simulink model "sensorMCUSlugsMKII"  (Simulink 6.6)
settings: Solver=FixedStepDiscrete  StartTime=0.0  StopTime=10.0  FixedStep=0.01  RelTol=1e-3
InitFcn:
  | mcuInit
values from neighbouring files (symbols this model uses):
  apSampleTime = 0.01    [mcuInit.m]
  T = 0.01    [mcuInit.m]
undefined symbols (not defined in the file or in its folder): accBiasRateLimit, accelXCutTemp, axTGain1, axTGain2, axTMean1, axTMean2, barAdjust, baroCutoff, baroCutTemp, baroOffset, baroScale, barTGain1, barTGain2, barTMean1, barTMean2, baseHeight, baseTemp, cubeAccelGain, cubeGyroGain, DiscIntNeverNeededParam, gaind, getCubeData, getGpsMainData, getMag, GS_location, gyroBiasRateLimit, lapseRate, lowRateSensorCutoff, magMeanTemp, magOffset, magScale, magTempK, mainSensorCutoff, maxDynPressure, param_acc, param_mag, pitAdjust, pitCutTemp, pitotOffset, pitotScale, pitTGain1, pitTGain2, pitTMean1, pitTMean2, polesd, powerOffset, powerScale, pressureSensorCutoff, q_quat, scheduleData, sensorMCUInit, spiSend, tempOffset, tempScale, u1, u2, updateAirData, updateAttitude, updateBias, updateDiagnosticFl ... (+14)
libraries: dsPICdrivers x38, simulink x14, aerolibutil x4, dspmtrx3 x2, aerolibconvert2 x2, SLUGS_Library x1
(part 2 of 4)

== system sensorMCUSlugsMKII/Position and Attitude Filter/GPS Update/Detect Change1 ==
  Data : Inport
  Abs1 : Abs  SampleTime=T
  Difference1 : simulink/Discrete/Difference  SystemSampleTime=-1  ICPrevInput=0.0  OutDataType=sfix(16)  OutScaling=2^-10  DoSatur=off
  Saturation1 : Saturate  UpperLimit=1  LowerLimit=0  SampleTime=T
  change? : Outport
  wires:
  Saturation1/1 -> change?/1
  Data/1 -> Difference1/1
  Abs1/1 -> Saturation1/1
  Difference1/1 -> Abs1/1

== system sensorMCUSlugsMKII/Position and Attitude Filter/GPS Update/Detect Change2 ==
  Data : Inport
  Abs1 : Abs  SampleTime=T
  Difference1 : simulink/Discrete/Difference  SystemSampleTime=-1  ICPrevInput=0.0  OutDataType=sfix(16)  OutScaling=2^-10  DoSatur=off
  Saturation1 : Saturate  UpperLimit=1  LowerLimit=0  SampleTime=T
  change? : Outport
  wires:
  Difference1/1 -> Abs1/1
  Abs1/1 -> Saturation1/1
  Data/1 -> Difference1/1
  Saturation1/1 -> change?/1

== system sensorMCUSlugsMKII/Position and Attitude Filter/Geod2LTP1/ECEF2LTP (UEN) ==
  ECEF coordinates : Inport
  "Long, Lat" : Inport  Port=2
  Deg2R : Gain  Gain=pi/180  SaturateOnIntegerOverflow=on
  Demux3 : Demux  Outputs=2
  From Body to Universal1 : Subsystem
  Product1 : Product  Multiplication=Matrix(*)  SaturateOnIntegerOverflow=on  InputSameDT=on
  Out : Outport
  wires:
  From Body to Universal1/1(DCM) -> Product1/1
  ECEF coordinates/1 -> Product1/2
  Deg2R/1 -> Demux3/1
  Demux3/1 -> From Body to Universal1/1(long)
  Demux3/2 -> From Body to Universal1/2(lat)
  Product1/1 -> Out/1
  "Long, Lat"/1 -> Deg2R/1

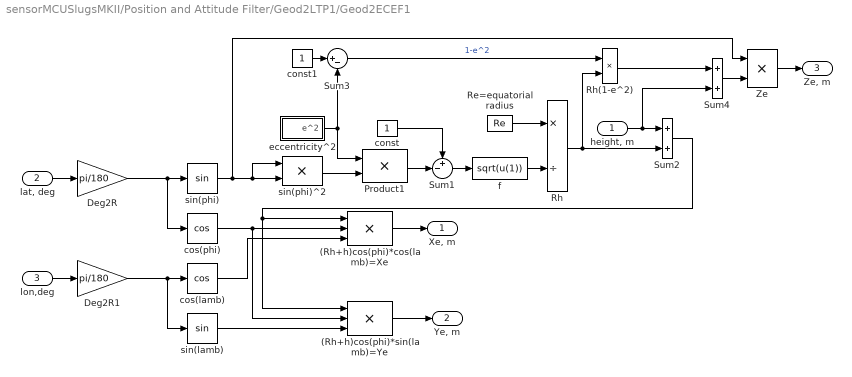
== system sensorMCUSlugsMKII/Position and Attitude Filter/Geod2LTP1/Geod2ECEF1 ==
  "height, m" : Inport
  "lat, deg" : Inport  Port=2
  lon,deg : Inport  Port=3
  (Rh+h)cos(phi)*cos(lamb)=Xe : Product  Inputs=3  OutDataTypeMode=single  SaturateOnIntegerOverflow=on  InputSameDT=on
  (Rh+h)cos(phi)*sin(lamb)=Ye : Product  Inputs=3  OutDataTypeMode=single  SaturateOnIntegerOverflow=on  InputSameDT=on
  Deg2R : Gain  Gain=pi/180  OutDataTypeMode=Specify via dialog  OutDataType=float('single')  SaturateOnIntegerOverflow=on
  Deg2R1 : Gain  Gain=pi/180  OutDataTypeMode=Specify via dialog  OutDataType=float('single')  SaturateOnIntegerOverflow=on
  Product1 : Product  SaturateOnIntegerOverflow=on  InputSameDT=on
  Re=equatorial radius : Constant  Value=Re  OutDataTypeMode=single
  Rh : Product  Inputs=*/  OutDataTypeMode=single  SaturateOnIntegerOverflow=on  InputSameDT=on
  Rh(1-e^2) : Product  OutDataTypeMode=single  SaturateOnIntegerOverflow=on  InputSameDT=on
  Sum1 : Sum  Inputs=+-|  SaturateOnIntegerOverflow=on  InputSameDT=on
  Sum2 : Sum  SaturateOnIntegerOverflow=on  InputSameDT=on
      settings: AttributesFormatString=Rh+h
  Sum3 : Sum  Inputs=|+-  SaturateOnIntegerOverflow=on  InputSameDT=on
  Sum4 : Sum  OutDataTypeMode=single  SaturateOnIntegerOverflow=on  InputSameDT=on
      settings: AttributesFormatString=(1-e^2)Rh+h
  Ze : Product  OutDataTypeMode=single  SaturateOnIntegerOverflow=on  InputSameDT=on
  const : Constant  OutDataTypeMode=single
  const1 : Constant  OutDataTypeMode=single
  cos(lamb) : Trigonometry  Operator=cos
  cos(phi) : Trigonometry  Operator=cos
  eccentricity^2 : Subsystem
  f : Fcn  Expr=sqrt(u(1))
  sin(lamb) : Trigonometry
  sin(phi) : Trigonometry
  sin(phi)^2 : Product  SaturateOnIntegerOverflow=on  InputSameDT=on
  "Xe, m " : Outport
  "Ye, m " : Outport  Port=2
  "Ze, m " : Outport  Port=3
  wires:
  (Rh+h)cos(phi)*sin(lamb)=Ye/1 -> "Ye, m "/1
  (Rh+h)cos(phi)*cos(lamb)=Xe/1 -> "Xe, m "/1
  Sum2/1 -> (Rh+h)cos(phi)*cos(lamb)=Xe/1, (Rh+h)cos(phi)*sin(lamb)=Ye/1
  Deg2R1/1 -> sin(lamb)/1, cos(lamb)/1
  Deg2R/1 -> sin(phi)/1, cos(phi)/1
  Ze/1 -> "Ze, m "/1
  sin(lamb)/1 -> (Rh+h)cos(phi)*sin(lamb)=Ye/3
  cos(lamb)/1 -> (Rh+h)cos(phi)*cos(lamb)=Xe/3
  cos(phi)/1 -> (Rh+h)cos(phi)*sin(lamb)=Ye/2, (Rh+h)cos(phi)*cos(lamb)=Xe/2
  lon,deg/1 -> Deg2R1/1
  Sum4/1 -> Ze/2
  Rh(1-e^2)/1 -> Sum4/1
  Sum3/1 -> Rh(1-e^2)/1  "1-e^2"
  const1/1 -> Sum3/1
  sin(phi)^2/1 -> Product1/2
  eccentricity^2/1(e^2) -> Sum3/2, Product1/1
  "height, m"/1 -> Sum2/1, Sum4/2
  const/1 -> Sum1/1
  Sum1/1 -> f/1
  Product1/1 -> Sum1/2
  Rh/1 -> Rh(1-e^2)/2, Sum2/2
  Re=equatorial radius/1 -> Rh/1
  f/1 -> Rh/2
  sin(phi)/1 -> Ze/1, sin(phi)^2/2, sin(phi)^2/1
  "lat, deg"/1 -> Deg2R/1

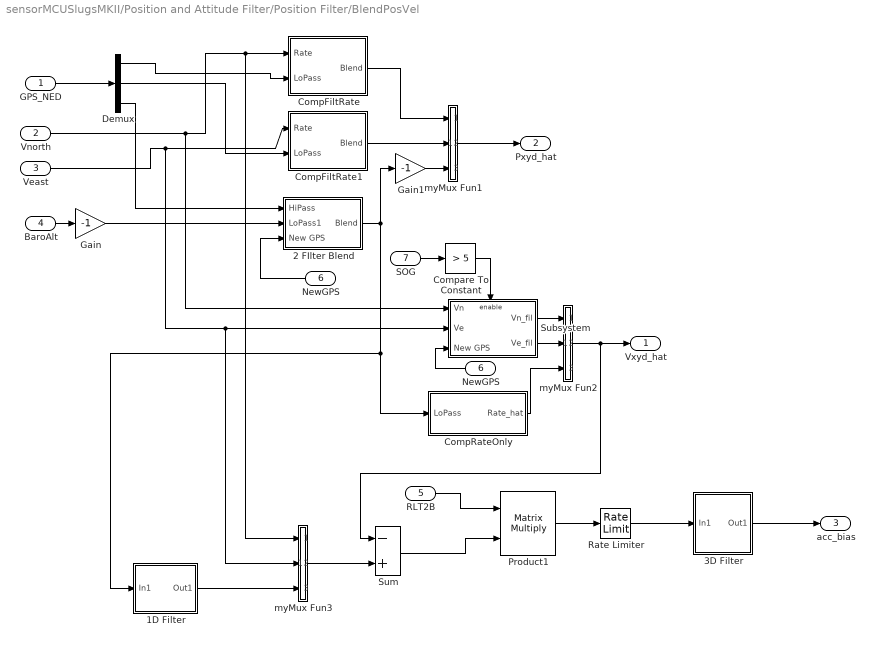
== system sensorMCUSlugsMKII/Position and Attitude Filter/Position Filter/BlendPosVel ==
  GPS_NED : Inport
  Vnorth : Inport  Port=2
  Veast : Inport  Port=3
  BaroAlt : Inport  Port=4
  RLT2B : Inport  Port=5
  NewGPS : Inport  Orientation=left  Port=6
  SOG : Inport  Port=7
  1D Filter : Subsystem  AncestorBlock=SLUGS_Library/Singnal Routing & Conditioning/3D Filter  RTWFcnName=TustinFilter3D  mask{zval=[0], pval=-50, kval=1, TSample=apSampleTime}
      mask prompts: zval "Zeros"; pval "Poles"; kval "Gains"; TSample "Sample Time"
      settings: RTWFcnNameOpts=User specified  RTWFileNameOpts=Use function name
      mask Display:
      | droots(zval,pval,kval)
      | port_label('input',1,'1D')
  2 FIlter Blend : Subsystem
  3D Filter : Subsystem  AncestorBlock=SLUGS_Library/Singnal Routing & Conditioning/3D Filter  RTWFcnName=TustinFilter3D  mask{zval=[], pval=[0], kval=1, TSample=0.01}
      mask prompts: zval "Zeros"; pval "Poles"; kval "Gains"; TSample "Sample Time"
      settings: RTWFcnNameOpts=User specified  RTWFileNameOpts=Use function name
      mask Display:
      | droots(zval,pval,kval)
      | port_label('input',1,'3D')
  CompFiltRate : Subsystem  mask{omega=xCutoff, T=apSampleTime}
      mask prompts: omega "Cutoff Freq (rad/sec)"; T "Sample Time"
  CompFiltRate1 : Subsystem  mask{omega=yCutoff, T=apSampleTime}
      mask prompts: omega "Cutoff Freq (rad/sec)"; T "Sample Time"
  CompRateOnly : Subsystem  mask{omega=vzCutoff, T=apSampleTime}
      mask prompts: omega "Cutoff Freq (rad/sec)"; T "Sample Time"
  Compare To Constant : simulink/Logic and Bit Operations/Compare To Constant  SystemSampleTime=-1  relop=>  const=5  LogicOutDataTypeMode=uint8  ZeroCross=off
  Demux : Demux  Outputs=3
  Gain : Gain  Gain=-1
  Gain1 : Gain  Gain=-1
  "NewGPS " : InportShadow  Orientation=left  Port=6  LatchByCopyingInsideSignal=off
  Product1 : Product  Multiplication=Matrix(*)  RndMeth=Zero
  Rate Limiter : RateLimiter  RisingSlewLimit=accBiasRateLimit  FallingSlewLimit=-accBiasRateLimit  SampleTimeMode=inherited
  Subsystem : Subsystem
  Sum : Sum  Inputs=-+  OutDataTypeMode=single
  myMux Fun1 : Stateflow chart
  myMux Fun2 : Stateflow chart
  myMux Fun3 : Stateflow chart
  Vxyd_hat : Outport
  Pxyd_hat : Outport  Port=2
  acc_bias : Outport  Port=3
  wires:
  Rate Limiter/1 -> 3D Filter/1(In1)
  3D Filter/1(Out1) -> acc_bias/1
  Sum/1 -> Product1/2
  myMux Fun3/1(y) -> Sum/2
  1D Filter/1(Out1) -> myMux Fun3/3(u3)
  Product1/1 -> Rate Limiter/1
  RLT2B/1 -> Product1/1
  CompRateOnly/1(Rate_hat) -> myMux Fun2/3(u3)
  Subsystem/2(Ve_fil) -> myMux Fun2/2(u2)
  Subsystem/1(Vn_fil) -> myMux Fun2/1(u1)
  Gain/1 -> 2 FIlter Blend/2(LoPass1)
  myMux Fun1/1(y) -> Pxyd_hat/1
  2 FIlter Blend/1(Blend) -> 1D Filter/1(In1), CompRateOnly/1(LoPass), Gain1/1
  CompFiltRate/1(Blend) -> myMux Fun1/1(u1)
  CompFiltRate1/1(Blend) -> myMux Fun1/2(u2)
  Demux/3 -> 2 FIlter Blend/1(HiPass)
  BaroAlt/1 -> Gain/1
  Demux/2 -> CompFiltRate1/2(LoPass)
  Demux/1 -> CompFiltRate/2(LoPass)
  Veast/1 -> myMux Fun3/2(u2), Subsystem/2(Ve), CompFiltRate1/1(Rate)
  Vnorth/1 -> CompFiltRate/1(Rate), myMux Fun3/1(u1), Subsystem/1(Vn)
  GPS_NED/1 -> Demux/1
  Gain1/1 -> myMux Fun1/3(u3)
  myMux Fun2/1(y) -> Vxyd_hat/1, Sum/1
  NewGPS/1 -> Subsystem/3(New GPS)
  Compare To Constant/1 -> Subsystem/Enable
  SOG/1 -> Compare To Constant/1
  "NewGPS "/1 -> 2 FIlter Blend/3(New GPS)

== system sensorMCUSlugsMKII/Sensor Data/Sensor Suite/Compute CPU Load ==
  Calculus Time Step : dsPICdrivers/OTHERS/Calculus Time Step  Tag=dsPIC_CalculusTimeStep  SampleTime=0.01  PR1chk=on
  Data Type Conversion1 : DataTypeConversion  OutDataTypeMode=single
  Data Type Conversion12 : DataTypeConversion  OutDataTypeMode=uint8
  Data Type Conversion2 : DataTypeConversion  OutDataTypeMode=single
  Divide : Product  Inputs=*/  OutDataTypeMode=double  OutScaling=2^-10
  Gain : Gain  Gain=100
  Rounding Function : Rounding
  Load (%) : Outport
  wires:
  Calculus Time Step/1 -> Data Type Conversion2/1
  Calculus Time Step/2 -> Data Type Conversion1/1
  Divide/1 -> Gain/1
  Rounding Function/1 -> Data Type Conversion12/1
  Data Type Conversion1/1 -> Divide/2
  Data Type Conversion2/1 -> Divide/1
  Data Type Conversion12/1 -> Load (%)/1
  Gain/1 -> Rounding Function/1

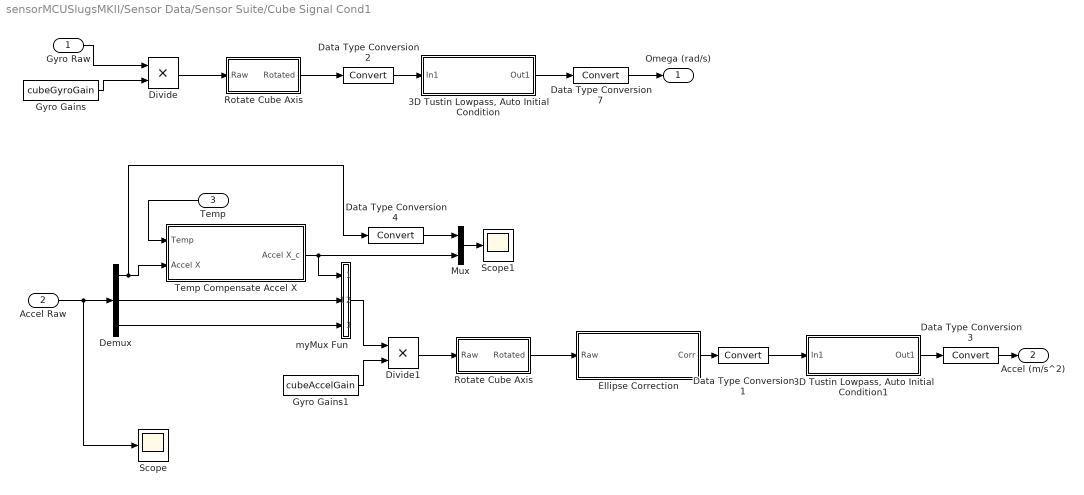
== system sensorMCUSlugsMKII/Sensor Data/Sensor Suite/Cube Signal Cond1 ==
  Gyro Raw : Inport
  Accel Raw : Inport  Port=2
  Temp : Inport  Orientation=left  Port=3
  "3D Tustin Lowpass, Auto Initial Condition" : Subsystem  mask(Tustin1stOrderLowpassAutoInitialCondition){f=mainSensorCutoff, T=T}
      mask prompts: f "Lowpass Frequency"; T "Sample Time"
      mask help: Takes a 3db rolloff frequency (in Hz, NOT radians/s) and a sample time. Performs a symbolic Tustin conversion and implements in a discrete filter. The initial output of the filter is set by the first sample.
      mask Help: Enter the desired 3db rolloff frequency in Hz and the sample time. Initial conditions are sampled automatically.
      mask Display: fprintf('%.2f Hz lowpass (3D)',f)
  "3D Tustin Lowpass, Auto Initial Condition1" : Subsystem  mask(Tustin1stOrderLowpassAutoInitialCondition){f=mainSensorCutoff, T=T}
      mask prompts: f "Lowpass Frequency"; T "Sample Time"
      mask help: Takes a 3db rolloff frequency (in Hz, NOT radians/s) and a sample time. Performs a symbolic Tustin conversion and implements in a discrete filter. The initial output of the filter is set by the first sample.
      mask Help: Enter the desired 3db rolloff frequency in Hz and the sample time. Initial conditions are sampled automatically.
      mask Display: fprintf('%.2f Hz lowpass (3D)',f)
  Data Type Conversion1 : DataTypeConversion  OutDataTypeMode=double
  Data Type Conversion2 : DataTypeConversion  OutDataTypeMode=double
  Data Type Conversion3 : DataTypeConversion  OutDataTypeMode=single
  Data Type Conversion4 : DataTypeConversion  OutDataTypeMode=single
  Data Type Conversion7 : DataTypeConversion  OutDataTypeMode=single
  Demux : Demux  Outputs=3
  Divide : Product  OutDataTypeMode=single  OutScaling=2^-10
  Divide1 : Product  OutDataTypeMode=single  OutScaling=2^-10
  Ellipse Correction : Subsystem  AncestorBlock=SLUGS_Library/Singnal Routing & Conditioning/Ellipse Correction  mask{param=param_acc}
      mask prompts: param "parameter (struct)"
      mask help: Applies the correction from the ellipse algorithm to the raw data being sent through the block. The block expects a 3x1 input vector, and will return a 3x1 output vector. The parameter constant should be a struct with param.xo .yo and .zo being the offsets, param.a .b and .c being the scale factors, and param.phi .rho and .lambda being the angle non-orthogonality (in degrees).
      mask Display:
      | text(0.2,0.85,'Ellipse Correction')
      | port_label('input',1,'RAW')
      | port_label('output',1,'CORR')
  Gyro Gains : Constant  Value=cubeGyroGain  OutDataTypeMode=single
  Gyro Gains1 : Constant  Value=cubeAccelGain  OutDataTypeMode=single
  Mux : Mux  Inputs=2
  Rotate Cube Axis : Subsystem
  "Rotate Cube Axis " : Subsystem
  Scope : Scope
      settings: YMin=-22.5  YMax=15  SaveName=ScopeData13
  Scope1 : Scope
      settings: YMin=-225  YMax=275  SaveName=ScopeData15
  Temp Compensate Accel X : Subsystem
  myMux Fun : Stateflow chart
  Omega (rad/s) : Outport
  Accel (m/s^2) : Outport  Port=2
  wires:
  Data Type Conversion4/1 -> Mux/1
  Mux/1 -> Scope1/1
  Demux/2 -> myMux Fun/2(u2)
  Gyro Gains/1 -> Divide/2
  Divide/1 -> Rotate Cube Axis/1(Raw)
  Divide1/1 -> "Rotate Cube Axis "/1(Raw)
  "Rotate Cube Axis "/1(Rotated) -> Ellipse Correction/1(Raw)
  Gyro Gains1/1 -> Divide1/2
  Gyro Raw/1 -> Divide/1
  Data Type Conversion2/1 -> "3D Tustin Lowpass, Auto Initial Condition"/1(In1)
  "3D Tustin Lowpass, Auto Initial Condition"/1(Out1) -> Data Type Conversion7/1
  Data Type Conversion7/1 -> Omega (rad/s)/1
  Rotate Cube Axis/1(Rotated) -> Data Type Conversion2/1
  Data Type Conversion1/1 -> "3D Tustin Lowpass, Auto Initial Condition1"/1(In1)
  "3D Tustin Lowpass, Auto Initial Condition1"/1(Out1) -> Data Type Conversion3/1
  Data Type Conversion3/1 -> Accel (m/s^2)/1
  Ellipse Correction/1(Corr) -> Data Type Conversion1/1
  Temp/1 -> Temp Compensate Accel X/1(Temp)
  Demux/3 -> myMux Fun/3(u3)
  Temp Compensate Accel X/1(Accel X_c) -> Mux/2, myMux Fun/1(u1)
  Demux/1 -> Data Type Conversion4/1, Temp Compensate Accel X/2(Accel X)
  Accel Raw/1 -> Scope/1, Demux/1
  myMux Fun/1(y) -> Divide1/1

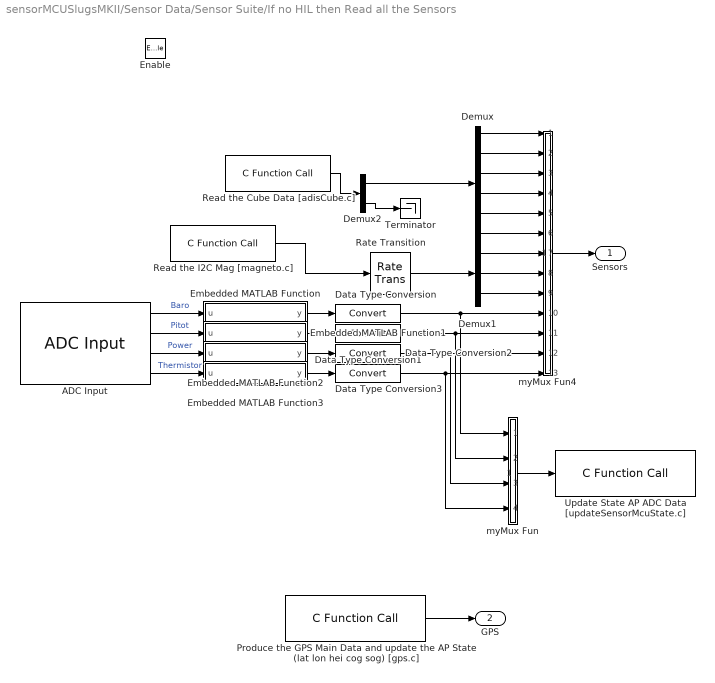
== system sensorMCUSlugsMKII/Sensor Data/Sensor Suite/If no HIL then Read all the Sensors ==
  Enable : EnablePort
  ADC Input : dsPICdrivers/Peripheral I//O/ADC Input  Tag=dsPIC_ADC  Priority=5  ADC_TYPE=12 bits  ADC_MODE=Continuous sampling & get last channel value  NbrSampleStep=4  VoltRefpopup="AVdd  -  AVss"  OutFormatBitspopup=0000 dddd dddd dddd : Integer  InterruptPriority=6  ANCHANNELS=[8 9 10 11]  MaxName=ANmax = 4095  Rin=200  ADCS=63  SAMC=31  Temperature=25  DMAChannel=1  SampleTime=.01  Status="OK  |  Tsmp=2.480e-005 |  T/Channel=3.600e-005 |  Tall=5.760e-004"  SSRC=auto convert
  Data Type Conversion{,1..3} (4 alike) : DataTypeConversion  OutDataTypeMode=int16
  Demux : Demux  Outputs=6
  Demux1 : Demux  Outputs=3
  Demux2 : Demux  Outputs=[6 1]
  Embedded MATLAB Function : Stateflow chart
  Embedded MATLAB Function1 : Stateflow chart
  Embedded MATLAB Function2 : Stateflow chart
  Embedded MATLAB Function3 : Stateflow chart
  Produce the GPS Main Data and update the AP State (lat lon hei cog sog) [gps.c] : dsPICdrivers/OTHERS/C Function Call  Tag=dsPIC_dsPIC_CFunctionCall  fctName='getGpsMainData'  INPUT_SIZE=1  INPUT1=--  INPUT2=--  INPUT3=--  OUTPUT_SIZE=5  OUTPUT1=real32  SampleTime=.01  InputType=[ ]  OutputType=[ 7 ]  FctDeclaration=extern void getGpsMainData(real32_T* y1);  FctCall=getGpsMainData(*%y1);  OrderingInOutPopup=None
  Rate Transition : RateTransition  OutPortSampleTime=0.01
  Read the Cube Data [adisCube.c] : dsPICdrivers/OTHERS/C Function Call  Tag=dsPIC_dsPIC_CFunctionCall  fctName='getCubeData'  INPUT_SIZE=1  INPUT1=--  INPUT2=--  INPUT3=--  OUTPUT_SIZE=7  OUTPUT1=int16  SampleTime=.01  InputType=[ ]  OutputType=[ 3 ]  FctDeclaration=extern void getCubeData(int16_T* y1);  FctCall=getCubeData(*%y1);  OrderingInOutPopup=None
  Read the I2C Mag [magneto.c] : dsPICdrivers/OTHERS/C Function Call  Tag=dsPIC_dsPIC_CFunctionCall  fctName='getMag'  INPUT_SIZE=1  INPUT1=--  INPUT2=--  INPUT3=--  OUTPUT_SIZE=3  OUTPUT1=int16  SampleTime=.01  InputType=[ ]  OutputType=[ 3 ]  FctDeclaration=extern void getMag(int16_T* y1);  FctCall=getMag(*%y1);  OrderingInOutPopup=None
  Terminator : Terminator
  Update State AP ADC Data [updateSensorMcuState.c] : dsPICdrivers/OTHERS/C Function Call  Tag=dsPIC_dsPIC_CFunctionCall  fctName='updateRawADCData'  INPUT_SIZE=4  INPUT1=int16  INPUT2=--  INPUT3=--  OUTPUT_SIZE=1  OUTPUT1=--  SampleTime=.01  InputType=[ 3 ]  OutputType=[ ]  FctDeclaration=extern void updateRawADCData(int16_T* u1);  FctCall=updateRawADCData(*%u1);  OrderingInOutPopup=None
  myMux Fun : Stateflow chart
  myMux Fun4 : Stateflow chart
  Sensors : Outport
  GPS : Outport  Port=2
  wires:
  myMux Fun4/1(y) -> Sensors/1
  Demux2/1 -> Demux/1
  Read the I2C Mag [magneto.c]/1 -> Rate Transition/1
  Demux/1 -> myMux Fun4/1(u1)
  Demux/2 -> myMux Fun4/2(u2)
  Demux/3 -> myMux Fun4/3(u3)
  Demux/4 -> myMux Fun4/4(u4)
  Demux/5 -> myMux Fun4/5(u5)
  Demux/6 -> myMux Fun4/6(u6)
  Demux1/1 -> myMux Fun4/7(u7)
  Demux1/2 -> myMux Fun4/8(u8)
  Demux1/3 -> myMux Fun4/9(u9)
  ADC Input/1 -> Embedded MATLAB Function/1(u)  "Baro"
  ADC Input/2 -> Embedded MATLAB Function1/1(u)  "Pitot"
  ADC Input/3 -> Embedded MATLAB Function2/1(u)  "Power"
  ADC Input/4 -> Embedded MATLAB Function3/1(u)  "Thermistor"
  myMux Fun/1(y) -> Update State AP ADC Data [updateSensorMcuState.c]/1
  Rate Transition/1 -> Demux1/1
  Data Type Conversion/1 -> myMux Fun4/10(u10), myMux Fun/1(u1)
  Data Type Conversion1/1 -> myMux Fun4/11(u11), myMux Fun/2(u2)
  Data Type Conversion2/1 -> myMux Fun4/12(u12), myMux Fun/3(u3)
  Data Type Conversion3/1 -> myMux Fun4/13(u13), myMux Fun/4(u4)
  Produce the GPS Main Data and update the AP State (lat lon hei cog sog) [gps.c]/1 -> GPS/1
  Embedded MATLAB Function/1(y) -> Data Type Conversion/1
  Embedded MATLAB Function1/1(y) -> Data Type Conversion1/1
  Embedded MATLAB Function2/1(y) -> Data Type Conversion2/1
  Embedded MATLAB Function3/1(y) -> Data Type Conversion3/1
  Read the Cube Data [adisCube.c]/1 -> Demux2/1
  Demux2/2 -> Terminator/1

== system sensorMCUSlugsMKII/Sensor Data/Sensor Suite/If no HIL then update Air Data ==
  AirData : Inport
  Enable : EnablePort
  Update the Air Calibrated Data [updateSensorMcuState.c] : dsPICdrivers/OTHERS/C Function Call  Tag=dsPIC_dsPIC_CFunctionCall  fctName='updateAirData'  INPUT_SIZE=3  INPUT1=real32  INPUT2=--  INPUT3=--  OUTPUT_SIZE=1  OUTPUT1=--  SampleTime=.01  InputType=[ 7 ]  OutputType=[ ]  FctDeclaration=extern void updateAirData(real32_T* u1);  FctCall=updateAirData(*%u1);  OrderingInOutPopup=None
  wires:
  AirData/1 -> Update the Air Calibrated Data [updateSensorMcuState.c]/1

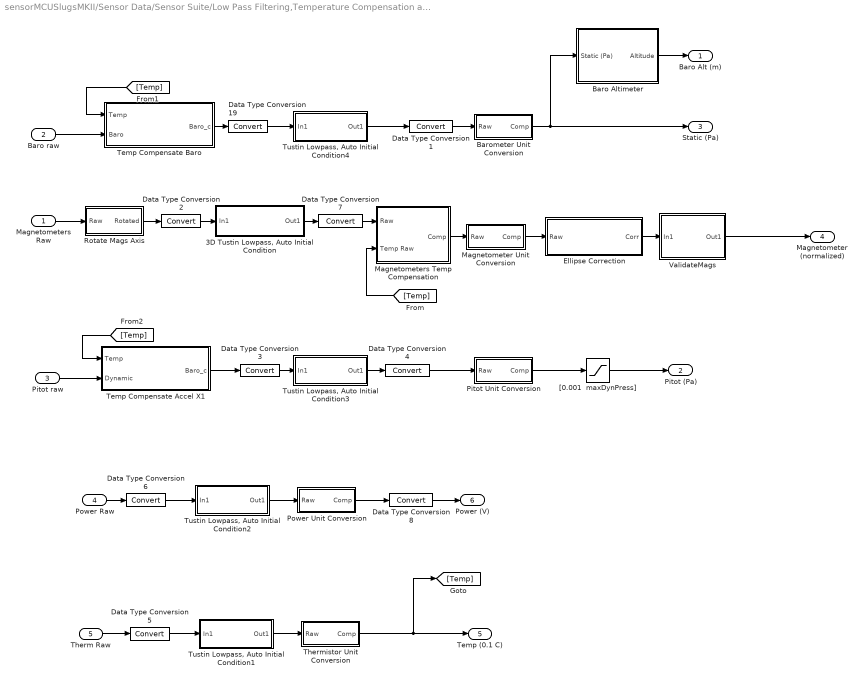
== system sensorMCUSlugsMKII/Sensor Data/Sensor Suite/Low Pass Filtering,Temperature Compensation and Calibration1 ==
  Magnetometers Raw : Inport
  Baro raw : Inport  Port=2
  Pitot raw : Inport  Port=3
  Power Raw : Inport  Port=4
  Therm Raw : Inport  Port=5
  "3D Tustin Lowpass, Auto Initial Condition" : Subsystem  mask(Tustin1stOrderLowpassAutoInitialCondition){f=mainSensorCutoff, T=T}
      mask prompts: f "Lowpass Frequency"; T "Sample Time"
      mask help: Takes a 3db rolloff frequency (in Hz, NOT radians/s) and a sample time. Performs a symbolic Tustin conversion and implements in a discrete filter. The initial output of the filter is set by the first sample.
      mask Help: Enter the desired 3db rolloff frequency in Hz and the sample time. Initial conditions are sampled automatically.
      mask Display: fprintf('%.2f Hz lowpass (3D)',f)
  Baro Altimeter : Subsystem
  Barometer Unit Conversion : Subsystem  mask{bias=baroOffset, gains=baroScale}
      mask prompts: bias "Initial Bias"; gains "Initial Gains"
      mask help: Convert Analog readings to units
  Data Type Conversion1 : DataTypeConversion  OutDataTypeMode=single
  Data Type Conversion{2..3,5..6,19} (5 alike) : DataTypeConversion  OutDataTypeMode=double
  Data Type Conversion4 : DataTypeConversion  OutDataTypeMode=single
  Data Type Conversion7 : DataTypeConversion  OutDataTypeMode=single
  Data Type Conversion8 : DataTypeConversion  OutDataTypeMode=uint16
  Ellipse Correction : Subsystem  AncestorBlock=SLUGS_Library/Singnal Routing & Conditioning/Ellipse Correction  mask{param=param_mag}
      mask prompts: param "parameter (struct)"
      mask help: Applies the correction from the ellipse algorithm to the raw data being sent through the block. The block expects a 3x1 input vector, and will return a 3x1 output vector. The parameter constant should be a struct with param.xo .yo and .zo being the offsets, param.a .b and .c being the scale factors, and param.phi .rho and .lambda being the angle non-orthogonality (in degrees).
      mask Display:
      | text(0.2,0.85,'Ellipse Correction')
      | port_label('input',1,'RAW')
      | port_label('output',1,'CORR')
  Magnetometer Unit Conversion : Subsystem  mask{bias=magOffset, gains=magScale}
      mask prompts: bias "Initial Bias"; gains "Initial Gains"
      mask help: Convert Analog readings to units
  Magnetometers Temp Compensation : Subsystem  mask{alpha=magTempK, tempMean=magMeanTemp}
      mask prompts: alpha "Tempearature Coeficient (K_t)"; tempMean "Calibration Temperature Mean (T_avg)"
      mask help:
      | This block implements a temperature compensation. It implmements the following equation:
      |
      | M_tc = M_raw - K_t(T - T_avg)
  Pitot Unit Conversion : Subsystem  mask{bias=pitotOffset, gains=pitotScale}
      mask prompts: bias "Initial Bias"; gains "Initial Gains"
      mask help: Convert Analog readings to units
  Power Unit Conversion : Subsystem  mask{bias=powerOffset, gains=powerScale}
      mask prompts: bias "Initial Bias"; gains "Initial Gains"
      mask help: Convert Analog readings to units
  Rotate Mags Axis : Subsystem
  Temp Compensate Accel X1 : Subsystem
  Temp Compensate Baro : Subsystem
  Thermistor Unit Conversion : Subsystem  mask{bias=tempOffset, gains=tempScale}
      mask prompts: bias "Initial Bias"; gains "Initial Gains"
      mask help: Convert Analog readings to units
  "Tustin Lowpass, Auto Initial Condition1" : Subsystem  mask(Tustin1stOrderLowpassAutoInitialCondition){f=lowRateSensorCutoff, T=T}
      mask prompts: f "Lowpass Frequency"; T "Sample Time"
      mask help: Takes a 3db rolloff frequency (in Hz, NOT radians/s) and a sample time. Performs a symbolic Tustin conversion and implements in a discrete filter. The initial output of the filter is set by the first sample.
      mask Help: Enter the desired 3db rolloff frequency in Hz and the sample time. Initial conditions are sampled automatically.
      mask Display: fprintf('%.2f Hz lowpass',f)
  "Tustin Lowpass, Auto Initial Condition2" : Subsystem  mask(Tustin1stOrderLowpassAutoInitialCondition){f=lowRateSensorCutoff, T=T}
      mask prompts: f "Lowpass Frequency"; T "Sample Time"
      mask help: Takes a 3db rolloff frequency (in Hz, NOT radians/s) and a sample time. Performs a symbolic Tustin conversion and implements in a discrete filter. The initial output of the filter is set by the first sample.
      mask Help: Enter the desired 3db rolloff frequency in Hz and the sample time. Initial conditions are sampled automatically.
      mask Display: fprintf('%.2f Hz lowpass',f)
  "Tustin Lowpass, Auto Initial Condition3" : Subsystem  mask(Tustin1stOrderLowpassAutoInitialCondition){f=pressureSensorCutoff, T=T}
      mask prompts: f "Lowpass Frequency"; T "Sample Time"
      mask help: Takes a 3db rolloff frequency (in Hz, NOT radians/s) and a sample time. Performs a symbolic Tustin conversion and implements in a discrete filter. The initial output of the filter is set by the first sample.
      mask Help: Enter the desired 3db rolloff frequency in Hz and the sample time. Initial conditions are sampled automatically.
      mask Display: fprintf('%.2f Hz lowpass',f)
  "Tustin Lowpass, Auto Initial Condition4" : Subsystem  mask(Tustin1stOrderLowpassAutoInitialCondition){f=pressureSensorCutoff, T=T}
      mask prompts: f "Lowpass Frequency"; T "Sample Time"
      mask help: Takes a 3db rolloff frequency (in Hz, NOT radians/s) and a sample time. Performs a symbolic Tustin conversion and implements in a discrete filter. The initial output of the filter is set by the first sample.
      mask Help: Enter the desired 3db rolloff frequency in Hz and the sample time. Initial conditions are sampled automatically.
      mask Display: fprintf('%.2f Hz lowpass',f)
  ValidateMags : Subsystem
  "[0.001  maxDynPress]" : Saturate  UpperLimit=maxDynPressure  LowerLimit=0.001
  Baro Alt (m) : Outport
  Pitot (Pa) : Outport  Port=2
  Static (Pa) : Outport  Port=3
  Magnetometer (normalized) : Outport  Port=4
  Temp (0.1 C) : Outport  Port=5
  Power (V) : Outport  Port=6
  wires:
  Data Type Conversion2/1 -> "3D Tustin Lowpass, Auto Initial Condition"/1(In1)
  "3D Tustin Lowpass, Auto Initial Condition"/1(Out1) -> Data Type Conversion7/1
  "Tustin Lowpass, Auto Initial Condition1"/1(Out1) -> Thermistor Unit Conversion/1(Raw)
  "[0.001  maxDynPress]"/1 -> Pitot (Pa)/1
  Data Type Conversion19/1 -> "Tustin Lowpass, Auto Initial Condition4"/1(In1)
  Data Type Conversion3/1 -> "Tustin Lowpass, Auto Initial Condition3"/1(In1)
  "Tustin Lowpass, Auto Initial Condition3"/1(Out1) -> Data Type Conversion4/1
  Data Type Conversion5/1 -> "Tustin Lowpass, Auto Initial Condition1"/1(In1)
  Therm Raw/1 -> Data Type Conversion5/1
  Barometer Unit Conversion/1(Comp) -> Static (Pa)/1, Baro Altimeter/1(Static (Pa))
  Magnetometers Raw/1 -> Rotate Mags Axis/1(Raw)
  Data Type Conversion4/1 -> Pitot Unit Conversion/1(Raw)
  Data Type Conversion7/1 -> Magnetometers Temp Compensation/1(Raw)
  Magnetometers Temp Compensation/1(Comp) -> Magnetometer Unit Conversion/1(Raw)
  [Temp] -> Magnetometers Temp Compensation/2(Temp Raw)
  "Tustin Lowpass, Auto Initial Condition4"/1(Out1) -> Data Type Conversion1/1
  Data Type Conversion1/1 -> Barometer Unit Conversion/1(Raw)
  Thermistor Unit Conversion/1(Comp) -> Temp (0.1 C)/1, [Temp]
  Data Type Conversion6/1 -> "Tustin Lowpass, Auto Initial Condition2"/1(In1)
  Power Raw/1 -> Data Type Conversion6/1
  "Tustin Lowpass, Auto Initial Condition2"/1(Out1) -> Power Unit Conversion/1(Raw)
  Data Type Conversion8/1 -> Power (V)/1
  Baro Altimeter/1(Altitude) -> Baro Alt (m)/1
  Pitot Unit Conversion/1(Comp) -> "[0.001  maxDynPress]"/1
  Power Unit Conversion/1(Comp) -> Data Type Conversion8/1
  Magnetometer Unit Conversion/1(Comp) -> Ellipse Correction/1(Raw)
  Rotate Mags Axis/1(Rotated) -> Data Type Conversion2/1
  Ellipse Correction/1(Corr) -> ValidateMags/1(In1)
  ValidateMags/1(Out1) -> Magnetometer (normalized)/1
  Temp Compensate Baro/1(Baro_c) -> Data Type Conversion19/1
  [Temp] -> Temp Compensate Baro/1(Temp)
  Baro raw/1 -> Temp Compensate Baro/2(Baro)
  [Temp] -> Temp Compensate Accel X1/1(Temp)
  Pitot raw/1 -> Temp Compensate Accel X1/2(Dynamic)
  Temp Compensate Accel X1/1(Baro_c) -> Data Type Conversion3/1

== system sensorMCUSlugsMKII/Position and Attitude Filter/Attitude Complimentary Filter COG/3D Filter/Filter1 ==
  In1 : Inport
  Discrete Zero-Pole : DiscreteZeroPole  Zeros=zerosd  Poles=polesd  Gain=gaind  SampleTime=SampleTime
  Out1 : Outport
  wires:
  Discrete Zero-Pole/1 -> Out1/1
  In1/1 -> Discrete Zero-Pole/1

== system sensorMCUSlugsMKII/Position and Attitude Filter/Attitude Complimentary Filter COG/3D Filter/Filter2 ==
  In1 : Inport
  Discrete Zero-Pole : DiscreteZeroPole  Zeros=zerosd  Poles=polesd  Gain=gaind  SampleTime=SampleTime
  Out1 : Outport
  wires:
  In1/1 -> Discrete Zero-Pole/1
  Discrete Zero-Pole/1 -> Out1/1

== system sensorMCUSlugsMKII/Position and Attitude Filter/Attitude Complimentary Filter COG/3D Filter/Filter3 ==
  In1 : Inport
  Discrete Zero-Pole : DiscreteZeroPole  Zeros=zerosd  Poles=polesd  Gain=gaind  SampleTime=SampleTime
  Out1 : Outport
  wires:
  Discrete Zero-Pole/1 -> Out1/1
  In1/1 -> Discrete Zero-Pole/1

== system sensorMCUSlugsMKII/Position and Attitude Filter/Attitude Complimentary Filter COG/Direction Cosine Matrix to Euler Angles/Subsystem1 ==
  u : Inport
  v : Inport  Port=2
  C Function Call : dsPICdrivers/OTHERS/C Function Call  Tag=dsPIC_dsPIC_CFunctionCall  fctName='myAtan2'  INPUT_SIZE=1  INPUT1=real32  INPUT2=real32  INPUT3=--  OUTPUT_SIZE=1  OUTPUT1=real32  SampleTime=-1  InputType=[ 7 7 ]  OutputType=[ 7 ]  FctDeclaration=extern real32_T myAtan2(real32_T u1, real32_T u2);  FctCall=%y1 = myAtan2(%u1, %u2);  OrderingInOutPopup=None
  atan2(x,y) : Outport
  wires:
  C Function Call/1 -> atan2(x,y)/1
  v/1 -> C Function Call/2
  u/1 -> C Function Call/1

== system sensorMCUSlugsMKII/Position and Attitude Filter/Attitude Complimentary Filter COG/Direction Cosine Matrix to Euler Angles/Subsystem2 ==
  u : Inport
  v : Inport  Port=2
  C Function Call : dsPICdrivers/OTHERS/C Function Call  Tag=dsPIC_dsPIC_CFunctionCall  fctName='myAtan2'  INPUT_SIZE=1  INPUT1=real32  INPUT2=real32  INPUT3=--  OUTPUT_SIZE=1  OUTPUT1=real32  SampleTime=-1  InputType=[ 7 7 ]  OutputType=[ 7 ]  FctDeclaration=extern real32_T myAtan2(real32_T u1, real32_T u2);  FctCall=%y1 = myAtan2(%u1, %u2);  OrderingInOutPopup=None
  atan2(x,y) : Outport
  wires:
  u/1 -> C Function Call/1
  v/1 -> C Function Call/2
  C Function Call/1 -> atan2(x,y)/1

== system sensorMCUSlugsMKII/Position and Attitude Filter/Attitude Complimentary Filter COG/Direction Cosine Matrix to Euler Angles/Subsystem3 ==
  x : Inport
  C Function Call : dsPICdrivers/OTHERS/C Function Call  Tag=dsPIC_dsPIC_CFunctionCall  fctName='myAsin'  INPUT_SIZE=1  INPUT1=real32  INPUT2=--  INPUT3=--  OUTPUT_SIZE=1  OUTPUT1=real32  SampleTime=-1  InputType=[ 7 ]  OutputType=[ 7 ]  FctDeclaration=extern real32_T myAsin(real32_T u1);  FctCall=%y1 = myAsin(%u1);  OrderingInOutPopup=None
  "[-1,1]" : Saturate  UpperLimit=0.9999  LowerLimit=-0.999
  asin(x) : Outport
  wires:
  C Function Call/1 -> asin(x)/1
  x/1 -> "[-1,1]"/1
  "[-1,1]"/1 -> C Function Call/1

== system sensorMCUSlugsMKII/Position and Attitude Filter/Attitude Complimentary Filter COG/Direction Cosine Matrix to Euler Angles/cos(phi)cos(theta) ==
  DCM : Inport
  Demux : Demux  Outputs=9
  Terminator{,1..7} (8 alike) : Terminator
  cos(phi)cos(theta) : Outport
  wires:
  Demux/4 -> Terminator/1
  Demux/3 -> Terminator1/1
  Demux/5 -> Terminator4/1
  Demux/2 -> Terminator3/1
  Demux/1 -> Terminator2/1
  DCM/1 -> Demux/1
  Demux/8 -> Terminator7/1
  Demux/6 -> Terminator5/1
  Demux/7 -> Terminator6/1
  Demux/9 -> cos(phi)cos(theta)/1

== system sensorMCUSlugsMKII/Position and Attitude Filter/Attitude Complimentary Filter COG/Direction Cosine Matrix to Euler Angles/cos(psi)cos(theta) ==
  DCM : Inport
  Demux : Demux  Outputs=9
  Terminator{,1..7} (8 alike) : Terminator
  cos(psi)cos(theta) : Outport
  wires:
  Demux/9 -> Terminator2/1
  Demux/7 -> Terminator6/1
  Demux/6 -> Terminator5/1
  Demux/8 -> Terminator7/1
  DCM/1 -> Demux/1
  Demux/1 -> cos(psi)cos(theta)/1
  Demux/2 -> Terminator3/1
  Demux/5 -> Terminator4/1
  Demux/3 -> Terminator1/1
  Demux/4 -> Terminator/1

== system sensorMCUSlugsMKII/Position and Attitude Filter/Attitude Complimentary Filter COG/Direction Cosine Matrix to Euler Angles/sin(phi)cos(theta) ==
  DCM : Inport
  Demux : Demux  Outputs=9
  Terminator{,1..7} (8 alike) : Terminator
  sin(phi)cos(theta) : Outport
  wires:
  Demux/9 -> Terminator7/1
  Demux/7 -> Terminator6/1
  Demux/6 -> Terminator5/1
  Demux/8 -> sin(phi)cos(theta)/1
  DCM/1 -> Demux/1
  Demux/1 -> Terminator2/1
  Demux/2 -> Terminator3/1
  Demux/5 -> Terminator4/1
  Demux/3 -> Terminator1/1
  Demux/4 -> Terminator/1

== system sensorMCUSlugsMKII/Position and Attitude Filter/Attitude Complimentary Filter COG/Direction Cosine Matrix to Euler Angles/sin(psi)cos(theta) ==
  DCM : Inport
  Demux : Demux  Outputs=9
  Terminator{,1..7} (8 alike) : Terminator
  sin(psi)cos(theta) : Outport
  wires:
  Demux/4 -> sin(psi)cos(theta)/1
  Demux/3 -> Terminator1/1
  Demux/5 -> Terminator4/1
  Demux/2 -> Terminator3/1
  Demux/1 -> Terminator2/1
  DCM/1 -> Demux/1
  Demux/8 -> Terminator/1
  Demux/6 -> Terminator5/1
  Demux/7 -> Terminator6/1
  Demux/9 -> Terminator7/1

== system sensorMCUSlugsMKII/Position and Attitude Filter/Attitude Complimentary Filter COG/Direction Cosine Matrix to Euler Angles/sin(theta) ==
  DCM : Inport
  Demux : Demux  Outputs=9
  Gain2 : Gain  Gain=-1  SaturateOnIntegerOverflow=on
  Terminator{,1..5,7..8} (8 alike) : Terminator
  sin(theta) : Outport
  wires:
  Gain2/1 -> sin(theta)/1
  Demux/4 -> Terminator/1
  Demux/3 -> Terminator1/1
  Demux/5 -> Terminator4/1
  Demux/2 -> Terminator3/1
  Demux/1 -> Terminator2/1
  DCM/1 -> Demux/1
  Demux/8 -> Terminator8/1
  Demux/6 -> Terminator5/1
  Demux/7 -> Gain2/1
  Demux/9 -> Terminator7/1

== system sensorMCUSlugsMKII/Position and Attitude Filter/Attitude Complimentary Filter COG/Normalize Vector1/Norm ==
  Vector : Inport
  Subsystem2 : Subsystem  AncestorBlock=SLUGS_Library/Subsystem1
  Subsystem3 : Subsystem  AncestorBlock=SLUGS_Library/Subsystem3
  Norm : Outport
  wires:
  Subsystem3/1(x dot y) -> Subsystem2/1(x)
  Vector/1 -> Subsystem3/2(y), Subsystem3/1(x)
  Subsystem2/1(sqrt(x)) -> Norm/1

== system sensorMCUSlugsMKII/Position and Attitude Filter/Attitude Complimentary Filter COG/Normalize Vector2/Norm ==
  Vector : Inport
  Subsystem2 : Subsystem  AncestorBlock=SLUGS_Library/Subsystem1
  Subsystem3 : Subsystem  AncestorBlock=SLUGS_Library/Subsystem3
  Norm : Outport
  wires:
  Subsystem2/1(sqrt(x)) -> Norm/1
  Vector/1 -> Subsystem3/1(x), Subsystem3/2(y)
  Subsystem3/1(x dot y) -> Subsystem2/1(x)

== system sensorMCUSlugsMKII/Position and Attitude Filter/Attitude Complimentary Filter COG/Quaternion Normalize/Quaternion Modulus ==
  q : Inport
  Quaternion Norm : aerolibutil/Quaternion Norm  SystemSampleTime=-1
  Subsystem1 : Subsystem  AncestorBlock=SLUGS_Library/Subsystem1
  |q| : Outport
  wires:
  Quaternion Norm/1 -> Subsystem1/1(x)
  q/1 -> Quaternion Norm/1
  Subsystem1/1(sqrt(x)) -> |q|/1

== system sensorMCUSlugsMKII/Position and Attitude Filter/Attitude Complimentary Filter COG/Quaternions to  Direction Cosine Matrix/A11 ==
  normal(q) : Inport
  Demux : Demux
  Product{,1..3} (4 alike) : Product  RndMeth=Zero
  Sum : Sum  Inputs=++--
  A11 : Outport
  wires:
  Sum/1 -> A11/1
  Demux/4 -> Product/2, Product/1
  Demux/3 -> Product1/2, Product1/1
  Demux/2 -> Product2/2, Product2/1
  Demux/1 -> Product3/2, Product3/1
  Product3/1 -> Sum/1
  Product2/1 -> Sum/2
  Product1/1 -> Sum/3
  Product/1 -> Sum/4
  normal(q)/1 -> Demux/1

== system sensorMCUSlugsMKII/Position and Attitude Filter/Attitude Complimentary Filter COG/Quaternions to  Direction Cosine Matrix/A12 ==
  normal(q) : Inport
  Demux : Demux
  Gain : Gain  Gain=2
  Product2 : Product  RndMeth=Zero
  Product3 : Product  RndMeth=Zero
  Sum : Sum  Inputs=|++
  A12 : Outport
  wires:
  Product2/1 -> Sum/2
  Product3/1 -> Sum/1
  Sum/1 -> Gain/1
  Demux/1 -> Product3/2
  Demux/2 -> Product2/1
  Demux/4 -> Product3/1
  Demux/3 -> Product2/2
  normal(q)/1 -> Demux/1
  Gain/1 -> A12/1

== system sensorMCUSlugsMKII/Position and Attitude Filter/Attitude Complimentary Filter COG/Quaternions to  Direction Cosine Matrix/A13 ==
  normal(q) : Inport
  Demux : Demux
  Gain : Gain  Gain=2
  Product1 : Product  RndMeth=Zero
  Product2 : Product  RndMeth=Zero
  Sum : Sum  Inputs=|-+
  A13 : Outport
  wires:
  Demux/1 -> Product1/1
  Product1/1 -> Sum/1
  Product2/1 -> Sum/2
  Demux/4 -> Product2/2
  Demux/2 -> Product2/1
  Demux/3 -> Product1/2
  normal(q)/1 -> Demux/1
  Gain/1 -> A13/1
  Sum/1 -> Gain/1

== system sensorMCUSlugsMKII/Position and Attitude Filter/Attitude Complimentary Filter COG/Quaternions to  Direction Cosine Matrix/A21 ==
  normal(q) : Inport
  Demux : Demux
  Gain : Gain  Gain=2
  Product2 : Product  RndMeth=Zero
  Product3 : Product  RndMeth=Zero
  Sum : Sum  Inputs=|-+
  A21 : Outport
  wires:
  Gain/1 -> A21/1
  normal(q)/1 -> Demux/1
  Demux/3 -> Product2/2
  Demux/4 -> Product3/1
  Demux/2 -> Product2/1
  Demux/1 -> Product3/2
  Sum/1 -> Gain/1
  Product3/1 -> Sum/1
  Product2/1 -> Sum/2

== system sensorMCUSlugsMKII/Position and Attitude Filter/Attitude Complimentary Filter COG/Quaternions to  Direction Cosine Matrix/A22 ==
  normal(q) : Inport
  Demux : Demux
  Product{,1..3} (4 alike) : Product  RndMeth=Zero
  Sum : Sum  Inputs=+-+-
  A22 : Outport
  wires:
  normal(q)/1 -> Demux/1
  Product/1 -> Sum/4
  Product1/1 -> Sum/3
  Product2/1 -> Sum/2
  Product3/1 -> Sum/1
  Demux/1 -> Product3/1, Product3/2
  Demux/2 -> Product2/1, Product2/2
  Demux/3 -> Product1/1, Product1/2
  Demux/4 -> Product/1, Product/2
  Sum/1 -> A22/1

== system sensorMCUSlugsMKII/Position and Attitude Filter/Attitude Complimentary Filter COG/Quaternions to  Direction Cosine Matrix/A23 ==
  normal(q) : Inport
  Demux : Demux
  Gain : Gain  Gain=2
  Product1 : Product  RndMeth=Zero
  Product2 : Product  RndMeth=Zero
  Sum : Sum  Inputs=|++
  A23 : Outport
  wires:
  Demux/4 -> Product2/2
  Product2/1 -> Sum/2
  Product1/1 -> Sum/1
  Sum/1 -> Gain/1
  Demux/1 -> Product1/1
  Demux/2 -> Product1/2
  Demux/3 -> Product2/1
  Gain/1 -> A23/1
  normal(q)/1 -> Demux/1

== system sensorMCUSlugsMKII/Position and Attitude Filter/Attitude Complimentary Filter COG/Quaternions to  Direction Cosine Matrix/A31 ==
  normal(q) : Inport
  Demux : Demux
  Gain : Gain  Gain=2
  Product1 : Product  RndMeth=Zero
  Product2 : Product  RndMeth=Zero
  Sum : Sum  Inputs=|++
  A31 : Outport
  wires:
  Sum/1 -> Gain/1
  Gain/1 -> A31/1
  normal(q)/1 -> Demux/1
  Demux/3 -> Product1/2
  Demux/2 -> Product2/1
  Demux/4 -> Product2/2
  Product2/1 -> Sum/2
  Product1/1 -> Sum/1
  Demux/1 -> Product1/1

== system sensorMCUSlugsMKII/Position and Attitude Filter/Attitude Complimentary Filter COG/Quaternions to  Direction Cosine Matrix/A32 ==
  normal(q) : Inport
  Demux : Demux
  Gain : Gain  Gain=2
  Product1 : Product  RndMeth=Zero
  Product2 : Product  RndMeth=Zero
  Sum : Sum  Inputs=|-+
  A32 : Outport
  wires:
  normal(q)/1 -> Demux/1
  Gain/1 -> A32/1
  Demux/3 -> Product2/1
  Demux/2 -> Product1/2
  Demux/1 -> Product1/1
  Sum/1 -> Gain/1
  Product1/1 -> Sum/1
  Product2/1 -> Sum/2
  Demux/4 -> Product2/2

== system sensorMCUSlugsMKII/Position and Attitude Filter/Attitude Complimentary Filter COG/Quaternions to  Direction Cosine Matrix/A33 ==
  normal(q) : Inport
  Demux : Demux
  Product{,1..3} (4 alike) : Product  RndMeth=Zero
  Sum : Sum  Inputs=+--+
  A33 : Outport
  wires:
  normal(q)/1 -> Demux/1
  Product/1 -> Sum/4
  Product1/1 -> Sum/3
  Product2/1 -> Sum/2
  Product3/1 -> Sum/1
  Demux/1 -> Product3/1, Product3/2
  Demux/2 -> Product2/1, Product2/2
  Demux/3 -> Product1/1, Product1/2
  Demux/4 -> Product/1, Product/2
  Sum/1 -> A33/1

== system sensorMCUSlugsMKII/Position and Attitude Filter/Attitude Complimentary Filter COG/Quaternions to  Direction Cosine Matrix/Create Transformation Matrix ==
  M11 : Inport
  M12 : Inport  Port=2
  M13 : Inport  Port=3
  M21 : Inport  Port=4
  M22 : Inport  Port=5
  M23 : Inport  Port=6
  M31 : Inport  Port=7
  M32 : Inport  Port=8
  M33 : Inport  Port=9
  Reshape (9) to [3x3] column-major : Reshape  OutputDimensionality=Customize  OutputDimensions=[3,3]
  myMux Fun1 : Stateflow chart
  Matrix : Outport
  wires:
  M33/1 -> myMux Fun1/9(u9)
  M23/1 -> myMux Fun1/8(u8)
  M13/1 -> myMux Fun1/7(u7)
  M32/1 -> myMux Fun1/6(u6)
  Reshape (9) to [3x3] column-major/1 -> Matrix/1
  M22/1 -> myMux Fun1/5(u5)
  M12/1 -> myMux Fun1/4(u4)
  M31/1 -> myMux Fun1/3(u3)
  M21/1 -> myMux Fun1/2(u2)
  M11/1 -> myMux Fun1/1(u1)
  myMux Fun1/1(y) -> Reshape (9) to [3x3] column-major/1

== system sensorMCUSlugsMKII/Position and Attitude Filter/Compute GS Location/Geod2ECEF1/eccentricity^2 ==
  " " : Product  OutDataTypeMode=single  SaturateOnIntegerOverflow=on  InputSameDT=on
  Re=equatorial radius1 : Constant  Value=Re  OutDataTypeMode=single
  Rp=polar radius : Constant  Value=Rp  OutDataTypeMode=single
  Sum5 : Sum  Inputs=|+-  SaturateOnIntegerOverflow=on  InputSameDT=on
  const2 : Constant  OutDataTypeMode=single
  e^1 : Product  Inputs=*/  OutDataTypeMode=single  SaturateOnIntegerOverflow=on  InputSameDT=on
  e^2 : Outport
  wires:
  Sum5/1 -> e^2/1
  " "/1 -> Sum5/2
  e^1/1 -> " "/1, " "/2
  const2/1 -> Sum5/1
  Rp=polar radius/1 -> e^1/1
  Re=equatorial radius1/1 -> e^1/2

== system sensorMCUSlugsMKII/Position and Attitude Filter/Geod2LTP1/ECEF2LTP (UEN)/From Body to Universal1 ==
  long : Inport
  lat : Inport  Port=2
  Mux : Mux  Inputs=2
  Reshape 9x1->3x1 : S-Function  FunctionName=sreshape  Parameters=OutputDimensionality, OutputDimensions  mask(Reshape){OutputDimensionality=Customize, OutputDimensions=[3,3]}
      mask prompts: OutputDimensionality "Output dimensionality:"; OutputDimensions "Output dimensions:"
      mask help:
      | Change the dimensions of a vector or matrix input signal. Output
      |  - a one-dimensional array (vector),
      |  - a column vector (Mx1 matrix),
      |  - a row vector (1xN matrix), or
      |  - a matrix or vector with specified dimensions, e.g., [M, N] or [W].
      mask init:
      | s = reshapemask(gcb,'init');
      mask StyleString: popup(1-D array|Column vector|Row vector|Customize),edit
      mask CallbackString: reshapemask(gcb,'cbDimensionality')|
      mask Display: disp('Reshape')
  Rotation Matrix from Long//Lat : Subsystem
      mask Type: Vector Transformation
      mask Description: Vector Transformation
      mask Display: disp('axis')
  DCM : Outport
  wires:
  Reshape 9x1->3x1/1 -> DCM/1
  Rotation Matrix from Long//Lat/1(DCM) -> Reshape 9x1->3x1/1
  Mux/1 -> Rotation Matrix from Long//Lat/1(long lat)
  long/1 -> Mux/1
  lat/1 -> Mux/2

== system sensorMCUSlugsMKII/Position and Attitude Filter/Geod2LTP1/Geod2ECEF1/eccentricity^2 ==
  " " : Product  OutDataTypeMode=single  SaturateOnIntegerOverflow=on  InputSameDT=on
  Re=equatorial radius1 : Constant  Value=Re  OutDataTypeMode=single
  Rp=polar radius : Constant  Value=Rp  OutDataTypeMode=single
  Sum5 : Sum  Inputs=|+-  SaturateOnIntegerOverflow=on  InputSameDT=on
  const2 : Constant  OutDataTypeMode=single
  e^1 : Product  Inputs=*/  OutDataTypeMode=single  SaturateOnIntegerOverflow=on  InputSameDT=on
  e^2 : Outport
  wires:
  Sum5/1 -> e^2/1
  " "/1 -> Sum5/2
  e^1/1 -> " "/1, " "/2
  const2/1 -> Sum5/1
  Rp=polar radius/1 -> e^1/1
  Re=equatorial radius1/1 -> e^1/2

== system sensorMCUSlugsMKII/Position and Attitude Filter/Position Filter/BlendPosVel/1D Filter ==
  In1 : Inport
  Data Type Conversion1 : DataTypeConversion  OutDataTypeMode=single
  Data Type Conversion2 : DataTypeConversion  OutDataTypeMode=double
  Filter2 : Subsystem  mask(DiscretizedZeroPole){Zeros=zval, Poles=pval, Gain=kval, AbsTol=auto, SampleTime=TSample, method=tustin, Wc=1}
      mask prompts: Zeros "Zeros (enter in s-main:)"; Poles "Poles (enter in s-domain:)"; Gain "Gain (enter in s-domain:)"; AbsTol "Absolute tolerance:"; SampleTime "Sample time:"; Wc "Critical Frequency (Hz):"
      mask help: Continuous mask uses c2d to transform parameters onto the Discrete Zero-Pole block inside.
      mask init: same as sensorMCUSlugsMKII/Position and Attitude Filter/Attitude Complimentary Filter COG/3D Filter/Filter1
      mask StyleString: edit,edit,edit,edit,edit,popup(zoh|foh|tustin|prewarp|matched),edit
      mask CallbackString: |||||hidecrit|
      mask Display:
      | droots(zeross,poless,gainss)
      | text( 0.5, 1.0, method, 'verticalAlignment','top')
  Out1 : Outport
  wires:
  Filter2/1(Out1) -> Data Type Conversion1/1
  In1/1 -> Data Type Conversion2/1
  Data Type Conversion2/1 -> Filter2/1(In1)
  Data Type Conversion1/1 -> Out1/1

== system sensorMCUSlugsMKII/Position and Attitude Filter/Position Filter/BlendPosVel/2 FIlter Blend ==
  HiPass : Inport
  LoPass1 : Inport  Port=2
  New GPS : Inport  Port=3
  1D Filter : Subsystem  AncestorBlock=SLUGS_Library/Singnal Routing & Conditioning/3D Filter  RTWFcnName=TustinFilter3D  mask{zval=[0], pval=-zCutoff, kval=1, TSample=apSampleTime}
      mask prompts: zval "Zeros"; pval "Poles"; kval "Gains"; TSample "Sample Time"
      settings: RTWFcnNameOpts=User specified  RTWFileNameOpts=Use function name
      mask Display:
      | droots(zval,pval,kval)
      | port_label('input',1,'1D')
  Constant1 : Constant  Value=baseHeight  OutDataTypeMode=single
  Embedded MATLAB Function3 : Stateflow chart
  Sum : Sum  OutDataTypeMode=single
  "Tustin Lowpass,  Auto Initial Condition4" : Subsystem  mask(Tustin1stOrderLowpassAutoInitialCondition){f=baroCutoff, T=T}
      mask prompts: f "Lowpass Frequency"; T "Sample Time"
      mask help: Takes a 3db rolloff frequency (in Hz, NOT radians/s) and a sample time. Performs a symbolic Tustin conversion and implements in a discrete filter. The initial output of the filter is set by the first sample.
      mask Help: Enter the desired 3db rolloff frequency in Hz and the sample time. Initial conditions are sampled automatically.
      mask Display: fprintf('%.2f Hz lowpass',f)
  Blend : Outport
  wires:
  LoPass1/1 -> "Tustin Lowpass,  Auto Initial Condition4"/1(In1)
  1D Filter/1(Out1) -> Sum/1
  "Tustin Lowpass,  Auto Initial Condition4"/1(Out1) -> Sum/2
  Sum/1 -> Blend/1
  New GPS/1 -> Embedded MATLAB Function3/2(NewGPS)
  HiPass/1 -> Embedded MATLAB Function3/1(gps_h)
  Embedded MATLAB Function3/1(h) -> 1D Filter/1(In1)
  Constant1/1 -> Embedded MATLAB Function3/3(baseHeight)

== system sensorMCUSlugsMKII/Position and Attitude Filter/Position Filter/BlendPosVel/3D Filter ==
  In1 : Inport
  Data Type Conversion1 : DataTypeConversion  OutDataTypeMode=single
  Data Type Conversion2 : DataTypeConversion  OutDataTypeMode=double
  Demux : Demux  Outputs=3
  Filter1 : Subsystem  mask(DiscretizedZeroPole){Zeros=zval, Poles=pval, Gain=kval, AbsTol=auto, SampleTime=TSample, method=tustin, Wc=1}
      mask prompts: Zeros "Zeros (enter in s-main:)"; Poles "Poles (enter in s-domain:)"; Gain "Gain (enter in s-domain:)"; AbsTol "Absolute tolerance:"; SampleTime "Sample time:"; Wc "Critical Frequency (Hz):"
      mask help: Continuous mask uses c2d to transform parameters onto the Discrete Zero-Pole block inside.
      mask init: same as sensorMCUSlugsMKII/Position and Attitude Filter/Attitude Complimentary Filter COG/3D Filter/Filter1
      mask StyleString: edit,edit,edit,edit,edit,popup(zoh|foh|tustin|prewarp|matched),edit
      mask CallbackString: |||||hidecrit|
      mask Display:
      | droots(zeross,poless,gainss)
      | text( 0.5, 1.0, method, 'verticalAlignment','top')
  Filter2 : Subsystem  mask(DiscretizedZeroPole){Zeros=zval, Poles=pval, Gain=kval, AbsTol=auto, SampleTime=TSample, method=tustin, Wc=1}
      mask prompts: Zeros "Zeros (enter in s-main:)"; Poles "Poles (enter in s-domain:)"; Gain "Gain (enter in s-domain:)"; AbsTol "Absolute tolerance:"; SampleTime "Sample time:"; Wc "Critical Frequency (Hz):"
      mask help: Continuous mask uses c2d to transform parameters onto the Discrete Zero-Pole block inside.
      mask init: same as sensorMCUSlugsMKII/Position and Attitude Filter/Attitude Complimentary Filter COG/3D Filter/Filter1
      mask StyleString: edit,edit,edit,edit,edit,popup(zoh|foh|tustin|prewarp|matched),edit
      mask CallbackString: |||||hidecrit|
      mask Display:
      | droots(zeross,poless,gainss)
      | text( 0.5, 1.0, method, 'verticalAlignment','top')
  Filter3 : Subsystem  mask(DiscretizedZeroPole){Zeros=zval, Poles=pval, Gain=kval, AbsTol=auto, SampleTime=TSample, method=tustin, Wc=1}
      mask prompts: Zeros "Zeros (enter in s-main:)"; Poles "Poles (enter in s-domain:)"; Gain "Gain (enter in s-domain:)"; AbsTol "Absolute tolerance:"; SampleTime "Sample time:"; Wc "Critical Frequency (Hz):"
      mask help: Continuous mask uses c2d to transform parameters onto the Discrete Zero-Pole block inside.
      mask init: same as sensorMCUSlugsMKII/Position and Attitude Filter/Attitude Complimentary Filter COG/3D Filter/Filter1
      mask StyleString: edit,edit,edit,edit,edit,popup(zoh|foh|tustin|prewarp|matched),edit
      mask CallbackString: |||||hidecrit|
      mask Display:
      | droots(zeross,poless,gainss)
      | text( 0.5, 1.0, method, 'verticalAlignment','top')
  myMux Fun1 : Stateflow chart
  Out1 : Outport
  wires:
  myMux Fun1/1(y) -> Data Type Conversion1/1
  In1/1 -> Data Type Conversion2/1
  Filter3/1(Out1) -> myMux Fun1/3(u3)
  Filter2/1(Out1) -> myMux Fun1/2(u2)
  Filter1/1(Out1) -> myMux Fun1/1(u1)
  Demux/3 -> Filter3/1(In1)
  Demux/2 -> Filter2/1(In1)
  Demux/1 -> Filter1/1(In1)
  Data Type Conversion2/1 -> Demux/1
  Data Type Conversion1/1 -> Out1/1

== system sensorMCUSlugsMKII/Position and Attitude Filter/Position Filter/BlendPosVel/CompFiltRate ==
  Rate : Inport
  LoPass : Inport  Port=2
  1D Filter1 : Subsystem  AncestorBlock=SLUGS_Library/Singnal Routing & Conditioning/3D Filter  RTWFcnName=TustinFilter3D  mask{zval=[], pval=[0], kval=1, TSample=T}
      mask prompts: zval "Zeros"; pval "Poles"; kval "Gains"; TSample "Sample Time"
      settings: RTWFcnNameOpts=User specified  RTWFileNameOpts=Use function name
      mask Display:
      | droots(zval,pval,kval)
      | port_label('input',1,'1D')
  Gain : Gain  Gain=omega
  Sum : Sum  Inputs=++|
  Sum1 : Sum  Inputs=|+-
  Unit Delay : UnitDelay  Orientation=left  SampleTime=T
  Blend : Outport
  wires:
  Unit Delay/1 -> Sum1/2
  LoPass/1 -> Sum1/1
  Sum1/1 -> Gain/1
  Gain/1 -> Sum/2
  Rate/1 -> Sum/1
  Sum/1 -> 1D Filter1/1(In1)
  1D Filter1/1(Out1) -> Unit Delay/1, Blend/1
